simulink model "Assembly_R_Simscape"  (R2022b)
settings: Solver=VariableStepAuto  StartTime=0.0  StopTime=10  RelTol=1e-3
model workspace: external: MATLAB File C:\Users\maie1\Desktop\xml_R\Assembly_R_DataFile1.m (data not in the file)
undefined symbols (not defined in the file or in its folder): smiData, X, Y, Z
libraries: sm_lib x116, nesl_utility x8, simulink_extras x4
(part 3 of 3)

== matlab function Assembly_R_Simscape/MATLAB Function4 ==
  data: q1_ik output; x input; q2_ik output; q3_ik output; q4_ik output
function [q1_ik,q2_ik,q3_ik,q4_ik]= inverse_kinematics_func(x) 
pos = [x(1);x(2);x(3)];
e = 10^(-2);
qo = [0;20;-90;-100];
%initially
counter = 0;  
%J_inv_mat = inverse_jacobian_matrix(qo(1),qo(2),qo(3),qo(4));
J_f =[0 -0.100455858004140 0 -0.129154364647580;-0.307273208117348 0 -0.254384439280606 0;0 -0.307273208117348 0 0.223701921588887];
J_inv_mat = pinv(J_f);
fwd_mat_value = forward_kinematics_func_num(qo(1),qo(2),qo(3),qo(4));
fwd_mat_value = fwd_mat_value - pos;
q_new = qo - (J_inv_mat*fwd_mat_value);
error = abs(fwd_mat_value);

  while(error(1)>=e || error(2)>=e || error(3)>=e)
      q_n = q_new;
      %J_inv_mat = inverse_jacobian_matrix(q_n(1),q_n(2),q_n(3),q_n(4));
      J1 = [(7*pi*sin((pi*q_n(1))/180)*sin((pi*q_n(2))/180))/90 + (37*pi*cos((pi*q_n(4))/180)*sin((pi*q_n(1))/180)*sin((pi*q_n(2))/180))/450,- (7*pi*cos((pi*q_n(1))/180)*cos((pi*q_n(2))/180))/90 - (37*pi*cos((pi*q_n(1))/180)*cos((pi*q_n(2))/180)*cos((pi*q_n(4))/180))/450, 0, (37*pi*cos((pi*q_n(1))/180)*sin((pi*q_n(2))/180)*sin((pi*q_n(4))/180))/450;
    - (7*pi*cos((pi*q_n(1))/180)*sin((pi*q_n(2))/180))/90 - (37*pi*cos((pi*q_n(1))/180)*cos((pi*q_n(4))/180)*sin((pi*q_n(2))/180))/450, - (7*pi*cos((pi*q_n(2))/180)*sin((pi*q_n(1))/180))/90 - (37*pi*cos((pi*q_n(2))/180)*cos((pi*q_n(4))/180)*sin((pi*q_n(1))/180))/450, 0, (37*pi*sin((pi*q_n(1))/180)*sin((pi*q_n(2))/180)*sin((pi*q_n(4))/180))/450;
    0,                                   - (7*pi*sin((pi*q_n(2))/180))/90 - (37*pi*cos((pi*q_n(4))/180)*sin((pi*q_n(2))/180))/450, 0,                 -(37*pi*cos((pi*q_n(2))/180)*sin((pi*q_n(4))/180))/450];
J2 = [(37*pi*cos((pi*q_n(2))/180)*sin((pi*q_n(1))/180)*sin((pi*q_n(3))/180)*sin((pi*q_n(4))/180))/450 - (37*pi*cos((pi*q_n(1))/180)*cos((pi*q_n(3))/180)*sin((pi*q_n(4))/180))/450, (37*pi*cos((pi*q_n(1))/180)*sin((pi*q_n(2))/180)*sin((pi*q_n(3))/180)*sin((pi*q_n(4))/180))/450,   (37*pi*sin((pi*q_n(1))/180)*sin((pi*q_n(3))/180)*sin((pi*q_n(4))/180))/450 - (37*pi*cos((pi*q_n(1))/180)*cos((pi*q_n(2))/180)*cos((pi*q_n(3))/180)*sin((pi*q_n(4))/180))/450, - (37*pi*cos((pi*q_n(3))/180)*cos((pi*q_n(4))/180)*sin((pi*q_n(1))/180))/450 - (37*pi*cos((pi*q_n(1))/180)*cos((pi*q_n(2))/180)*cos((pi*q_n(4))/180)*sin((pi*q_n(3))/180))/450;
    - (37*pi*cos((pi*q_n(3))/180)*sin((pi*q_n(1))/180)*sin((pi*q_n(4))/180))/450 - (37*pi*cos((pi*q_n(1))/180)*cos((pi*q_n(2))/180)*sin((pi*q_n(3))/180)*sin((pi*q_n(4))/180))/450, (37*pi*sin((pi*q_n(1))/180)*sin((pi*q_n(2))/180)*sin((pi*q_n(3))/180)*sin((pi*q_n(4))/180))/450, - (37*pi*cos((pi*q_n(1))/180)*sin((pi*q_n(3))/180)*sin((pi*q_n(4))/180))/450 - (37*pi*cos((pi*q_n(2))/180)*cos((pi*q_n(3))/180)*sin((pi*q_n(1))/180)*sin((pi*q_n(4))/180))/450,   (37*pi*cos((pi*q_n(1))/180)*cos((pi*q_n(3))/180)*cos((pi*q_n(4))/180))/450 - (37*pi*cos((pi*q_n(2))/180)*cos((pi*q_n(4))/180)*sin((pi*q_n(1))/180)*sin((pi*q_n(3))/180))/450;
    0,                 -(37*pi*cos((pi*q_n(2))/180)*sin((pi*q_n(3))/180)*sin((pi*q_n(4))/180))/450,                                                                                    -(37*pi*cos((pi*q_n(3))/180)*sin((pi*q_n(2))/180)*sin((pi*q_n(4))/180))/450,                                                                                    -(37*pi*cos((pi*q_n(4))/180)*sin((pi*q_n(2))/180)*sin((pi*q_n(3))/180))/450];

J_f = J1+J2;
J_inv_mat = pinv(J_f);
      fwd_mat_value = forward_kinematics_func_num(q_n(1),q_n(2),q_n(3),q_n(4));
      fwd_mat_value = fwd_mat_value - pos;
      q_new = q_n - J_inv_mat*fwd_mat_value;
      error = abs(fwd_mat_value);
      counter=counter+1;
  end
  q1_ik = q_new(1);
  q2_ik = q_new(2);
  q3_ik = q_new(3);
  q4_ik = q_new(4);
end

== matlab function Assembly_R_Simscape/MATLAB Function5 ==
  data: Ts input; Task_Space output
function Task_Space = task_traj(Ts)
if(Ts<=5)
    Task_Space = [-7.774-2.5952*Ts;0;17];
else
    Task_Space = [-33.726+2.5952*Ts;0;17];
end
